simulink model "linear_controller"  (R2023b)
settings: Solver=VariableStepAuto  StartTime=0.0  StopTime=10.0  RelTol=1e-3
undefined symbols (not defined in the file or in its folder): op, u0
settings Model: Creator=fabioschneider  LastModifiedBy=fabioschneider

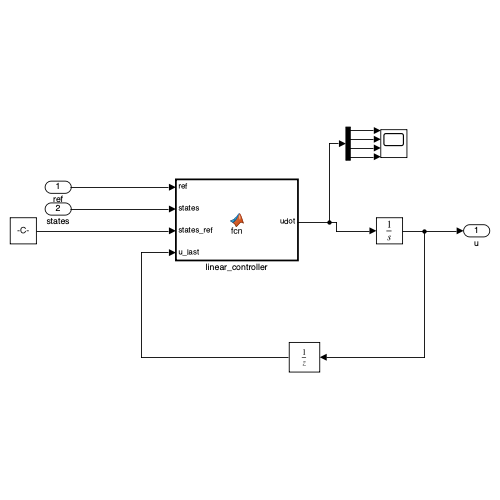
[thumbnail: Simulink's stored preview of the top-level diagram]
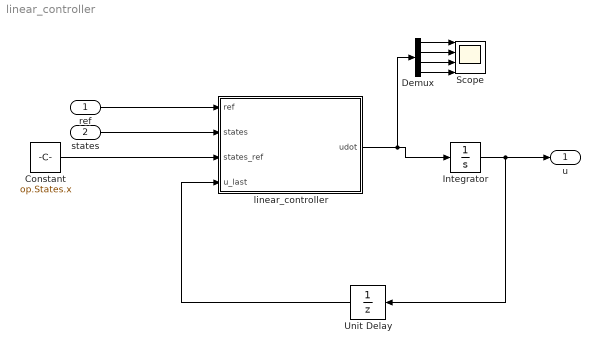
== system linear_controller ==
  ref : Inport  PortDimensions=[4;1]
  states : Inport  Port=2  PortDimensions=[9,1]
  Constant : Constant  Value=op.States.x
  Demux : Demux
  Integrator : Integrator  InitialCondition=op.Inputs.u
  Scope : Scope  NumInputPorts=4
  Unit Delay : UnitDelay  InitialCondition=u0  SampleTime=-1  HasFrameUpgradeWarning=on
  linear_controller : MATLAB Function  TreatAsAtomicUnit=on
  u : Outport
  wires:
  linear_controller/1(udot) -> Demux/1, Integrator/1
  Constant/1 -> linear_controller/3(states_ref)
  ref/1 -> linear_controller/1(ref)
  states/1 -> linear_controller/2(states)
  Integrator/1 -> Unit Delay/1, u/1
  Unit Delay/1 -> linear_controller/4(u_last)
  Demux/1 -> Scope/1
  Demux/2 -> Scope/2
  Demux/3 -> Scope/3
  Demux/4 -> Scope/4

== matlab function linear_controller/linear_controller ==
  data: ref input; udot output; states input; states_ref input; K parameter; u_last input
function udot = fcn(ref, states, states_ref, K, u_last)

udot = linear_controller_law(ref, states, states_ref, K, u_last);
